simulink model "AVR_library"  (R2019b)
settings: Solver=VariableStepAuto  StartTime=0.0  StopTime=10.0  RelTol=1e-3
undefined symbols (not defined in the file or in its folder): dyn, gcbh, j, sps_rtmsupport, Tb1, Tc1
libraries: simulink x5, spsST2AModel x4, modelLibrary x3
settings Model: Creator=gdudgeon  LastModifiedBy=gdudgeon
settings SFSimCC: CustomCodeUndefinedFunction=UseInterfaceOnly

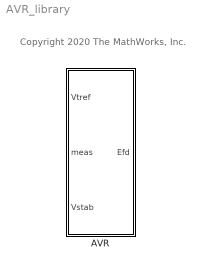
== system AVR_library ==
  note: Copyright 2020 The MathWorks, Inc.
  AVR : Subsystem  VariantControlMode=Label  Variant=on  LabelModeActiveChoice=Variant1
      settings: AttributesFormatString=%<BlockChoice>

== system AVR_library/AVR ==
  Vtref : Inport
  meas : Inport  Port=2
  Vstab : Inport  Port=3
  REXS : Subsystem  VariantControl=Variant1  mask{p=dyn.rexs_102_GAS}
      mask prompts: p "Parameters"
      mask DialogControl DescGroupVar Prompt: REXS
  ST1A : Subsystem  VariantControl=Variant2  mask{p=dyn.esst1a_102_HYDRO}
      mask prompts: p "Parameters"
      mask DialogControl DescGroupVar Prompt: ST1A
  ST4B : Subsystem  VariantControl=Variant3  mask{p=dyn.esst4b_102_STEAM}
      mask prompts: p "Parameters"
      mask DialogControl DescGroupVar Prompt: ST4B
  Efd : Outport  VectorParamsAs1DForOutWhenUnconnected=off

== system AVR_library/AVR/REXS ==
  Vtref : Inport
  meas : Inport  Port=2
  Vstab : Inport  Port=3
  Bus Selector1 : BusSelector  OutputSignals="dq0 components.Stator voltage  vd (pu),dq0 components.Stator voltage  vq (pu),dq0 components.Stator current  id (pu),dq0 components.Stator current  iq (pu),dq0 components.Field current  ifd (pu)"
  Euclidian Norm3 : Subsystem
  Euclidian Norm4 : Subsystem
  "Rotating Excitation System (Continuous) " : Subsystem  mask(PSS1A - Single Input Power System Stabilizer){Tr=p.tr, Kvp=p.kvp, Kvi=p.kvi, Vimax=p.vimax, Ta=p.ta, Tb=[p.tb1 p.tb2], Tc=[p.tc1 p.tc2], Vrrange=[p.vrmin p.vrmax], Kf=p.kf, Tf=p.tf, Tfll=[p.tf1 p.tf2], Fbf=p.fbf, Kip=p.kip, Kii=p.kii, Tp=p.tp, Kh=p.kh, Ke=p.ke, Te=p.te, Vfrange=[p.vfmin p.vfmax], Kc=p.kc, Kd=p.kd, E=[p.e1 p.e2], Se=[p.se1 p.se2], Xc=p.xc, Vcmax=p.vcmax, Kefd=p.kefd}
      mask prompts: Tr "Tr, Voltage Transducer Time Constant [s]"; Kvp "Kvp, Proportional Gain"; Kvi "Kvi, Integral Gain"; Vimax "Vimax, Input Limit [pu]"; Ta "Ta, Time Constant [s]"; Tb "Tb, Lag Time Constants [s]"; Tc "Tc, Lead Time Constants [s]"; Vrrange "[Vrmin Vrmax], Output Range [pu]"; Kf "Kf, Rate Gain"; Tf "Tf, Rate Time Constant [s]"; Tfll "[Tf1 Tf2], Lead/lag Contants [s]"; Fbf "Fbf, Feedback Signal Fl"; Kip "Kip, Regulator Proportional Gain"; Kii "Kii, Regulator Inegral Gain"; Tp "Tp, Bridge Time Constant [s]"; Kh "Kh, Voltage Controller Gain"; Ke "Ke, Exciter Proportional Constant"; Te "Te, Exciter Time Constant [s]"; Vfrange "[Vfmin Vfmax], Field Current Bounds [pu]"; Kc "Kc, Rectifier Regulation Factor [pu]"; Kd "Kd, Exciter Regulation Factor [pu]"; E "[E1 E2], Field Voltage Value Saturation"; Se "[Se1 Se2], Saturation Factor"; Xc "Xc,  Compounding Reactance [pu]"; Vcmax "Vcmax, Maximum Compounding Voltage [pu]"; Kefd "Kefd, Field Voltage Feedback"
      mask init:
      | % Extract Parameters
      | Tb1 = Tb(1);        Tb2 = Tb(2);
      | Tc1 = Tc(1);        Tc2 = Tc(2);
      | Tf1 = Tfll(1);      Tf2 = Tfll(2);
      | Vrmin = Vrrange(1); Vrmax = Vrrange(2);
      | Vfmin = Vfrange(1); Vfmax = Vfrange(2);
      mask DialogControl Container9 Prompt: Voltage Regulator
      mask DialogControl Container11 Prompt: Feedback Dynamics
      mask DialogControl Container25 Prompt: Field Current Regulator
      mask DialogControl Container29 Prompt: Rotating Exciter
      mask Display:
      | port_label('input',1,'Vref');
      | port_label('input',2,'Vt');
      | port_label('input',3,'It');
      | port_label('input',4,'Ifd');
      | port_label('input',5,'Vstab');
      | port_label('output',1,'Efd');
      | 
      | color('blue');disp('AVR/Exciter')
  Efd : Outport  VectorParamsAs1DForOutWhenUnconnected=off
  wires:
  meas/1 -> Bus Selector1/1
  "Rotating Excitation System (Continuous) "/1(Efd) -> Efd/1
  Bus Selector1/5 -> "Rotating Excitation System (Continuous) "/4(Ifd)  "<Field current  ifd (pu)>"
  Euclidian Norm3/1(y) -> "Rotating Excitation System (Continuous) "/2(Vt)  "Vt"
  Bus Selector1/2 -> Euclidian Norm3/2(u2)  "<Stator voltage  vq (pu)>"
  Bus Selector1/4 -> Euclidian Norm4/2(u2)  "<Stator current  iq (pu)>"
  Euclidian Norm4/1(y) -> "Rotating Excitation System (Continuous) "/3(It)  "It"
  Bus Selector1/3 -> Euclidian Norm4/1(u1)  "<Stator current  id (pu)>"
  Vtref/1 -> "Rotating Excitation System (Continuous) "/1(Vref)
  Bus Selector1/1 -> Euclidian Norm3/1(u1)  "<Stator voltage  vd (pu)>"
  Vstab/1 -> "Rotating Excitation System (Continuous) "/5(Vstab)

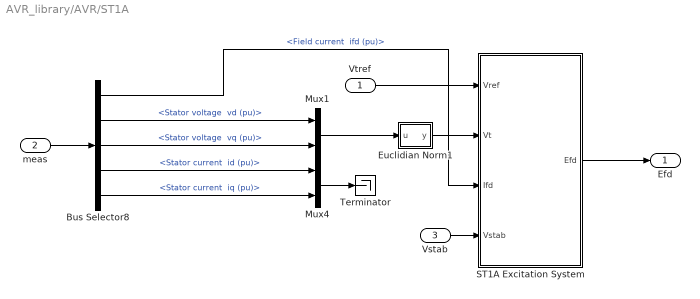
== system AVR_library/AVR/ST1A ==
  Vtref : Inport
  meas : Inport  Port=2
  Vstab : Inport  Port=3
  Bus Selector8 : BusSelector  OutputSignals="dq0 components.Field current  ifd (pu),dq0 components.Stator voltage  vd (pu),dq0 components.Stator voltage  vq (pu),dq0 components.Stator current  id (pu),dq0 components.Stator current  iq (pu)"
  Euclidian Norm1 : Subsystem
  Mux1 : Mux  Inputs=2
  Mux4 : Mux  Inputs=2
  ST1A Excitation System : Subsystem  DialogController=POWERSYS.PowerSysDialog  LoadFcn=sps_rtmsupport('LoadFcn', gcbh);  StartFcn=sps_rtmsupport('StartFcn', gcbh);  StopFcn=sps_rtmsupport('StopFcn', gcbh);  mask(ST1A Excitation System){Tr=20e-3, KaTa=[p.ka p.ta], VIminmax=[p.vimin p.vimax], VAminmax=[p.vamin p.vamax], VRminmax=[p.vrmin p.vrmax], KfTf=[p.kf p.tf], TbTc=[p.tb p.tc p.tb1 p.tc1], KLR=p.klr, ILR=p.ilr, Kc=p.kc, v0=[1 1], TsBlock=0}
      mask prompts: Tr "Low-pass filter time constant Tr(s):"; KaTa "Voltage regulator gain and time constant [Ka Ta(s)]:"; VIminmax "Voltage regulator input limits [VImin(pu) VImax(pu)]:"; VAminmax "Voltage regulator internal limits [VAmin(pu) VAmax(pu)]:"; VRminmax "Voltage regulator output limits [VRmin(pu) VRmax(pu)]:"; KfTf "Damping filter gain and time constant [Kf Tf(s)]:"; TbTc "Transient gain reduction lead and lag time constants [Tb(s) Tc(s) Tb1(s) Tc1(s)]:"; KLR "Exciter output current limiter gain KLR(pu):"; ILR "Exciter output current limit reference ILR(pu):"; Kc "Rectifier loading factor Kc(pu):"; v0 "Initial values of terminal voltage and field voltage [Vt0(pu) Efd0(pu)]:"; TsBlock "Sample time:"
      mask help: Implements a synchronous machine voltage regulator and exciter based on the IEEE type ST1A excitation system model. The output is the field voltage to apply to the Vf input of a Synchronous Machine block. Inputs and output are in p.u.
      mask init:
      | Ka = KaTa(1);
      | Ta = KaTa(2);
      | 
      | Kf = KfTf(1);
      | Tf = KfTf(2);
      | 
      | Tb = TbTc(1);
      | Tc = TbTc(2);
      settings: CopyFcn=sps_rtmsupport('CopyFcn', gcbh);  DeleteFcn=sps_rtmsupport('DeleteFcn', gcbh);  UndoDeleteFcn=sps_rtmsupport('UndoDeleteFcn', gcbh);  ModelCloseFcn=sps_rtmsupport('ModelCloseFcn', gcbh);  PreSaveFcn=sps_rtmsupport('PreSaveFcn', gcbh);  PostSaveFcn=sps_rtmsupport('PostSaveFcn', gcbh);  NameChangeFcn=sps_rtmsupport('NameChangeFcn', gcbh);  PreCopyFcn=sps_rtmsupport('PreCopyFcn', gcbh);  OpenFcn=sps_rtmsupport('OpenFcn', gcbh, []);  CloseFcn=sps_rtmsupport('CloseFcn', gcbh);  PreDeleteFcn=sps_rtmsupport('PreDeleteFcn', gcbh);
      mask Help: helpview(psbhelp);
      mask DialogControl ParameterTabVar0 Prompt: Controllers
      mask DialogControl ParameterTabVar01 Prompt: Exciter and Rectifier
      mask DialogControl ParameterTabVar012 Prompt: Initial Values
      mask Display: color('blue');disp('ST1A')
  Terminator : Terminator
  Efd : Outport  VectorParamsAs1DForOutWhenUnconnected=off
  wires:
  Mux4/1 -> Terminator/1
  ST1A Excitation System/1(Efd) -> Efd/1
  Vstab/1 -> ST1A Excitation System/4(Vstab)
  Bus Selector8/1 -> ST1A Excitation System/3(Ifd)  "<Field current  ifd (pu)>"
  Vtref/1 -> ST1A Excitation System/1(Vref)
  Bus Selector8/5 -> Mux4/2  "<Stator current  iq (pu)>"
  Bus Selector8/4 -> Mux4/1  "<Stator current  id (pu)>"
  meas/1 -> Bus Selector8/1
  Euclidian Norm1/1(y) -> ST1A Excitation System/2(Vt)
  Bus Selector8/2 -> Mux1/1  "<Stator voltage  vd (pu)>"
  Bus Selector8/3 -> Mux1/2  "<Stator voltage  vq (pu)>"
  Mux1/1 -> Euclidian Norm1/1(u)

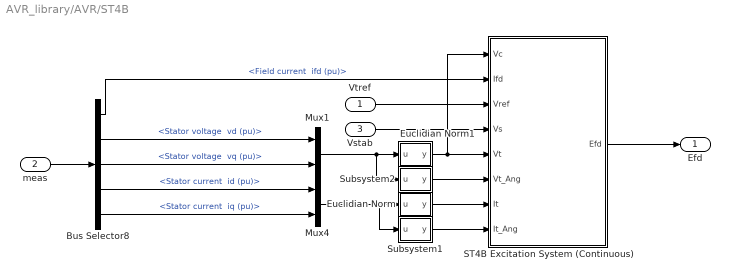
== system AVR_library/AVR/ST4B ==
  Vtref : Inport
  meas : Inport  Port=2
  Vstab : Inport  Port=3
  Bus Selector8 : BusSelector  OutputSignals="dq0 components.Field current  ifd (pu),dq0 components.Stator voltage  vd (pu),dq0 components.Stator voltage  vq (pu),dq0 components.Stator current  id (pu),dq0 components.Stator current  iq (pu)"
  Euclidian Norm : Subsystem
  Euclidian Norm1 : Subsystem
  Mux1 : Mux  Inputs=2
  Mux4 : Mux  Inputs=2
  ST4B Excitation System (Continuous) : Subsystem  mask(ST4B Excitation System){Tr=p.tr, Kpr=p.kpr, Kir=p.kir, Ta=p.ta, Vrmax=p.vrmax, Vrmin=p.vrmin, Kpm=p.kpm, Kim=p.kim, Kg=p.kg, Vmmin=p.vmmin, Vmmax=p.vmmax, Vgmax=p.vgmax, Kp=p.kp, Ki=p.ki, Angp=p.angp, Kc=p.kc, Xl=p.xl, Vbmax=p.vbmax}
      mask prompts: Tr "Voltage Transducer Time (Tr)"; Kpr "AVR Proportional Gain (Kpr)"; Kir "AVR Integral Gain (Kir)"; Ta "AVR Time Constant (Ta) [sec]"; Vrmax "Maximum AVR Output (Vrmax)"; Vrmin "Minimum AVR Output (Vrmin)"; Kpm "Inner Loop Regulator P Gain (Kpm)"; Kim "Inner Loop Regulator I gain (Kim)"; Kg "Inner Loop Feedback Gain (Kg)"; Vmmin "Inner Loop Regulator Min Output (Vmmin)"; Vmmax "Inner Loop Regulator Max Output (Vmmax)"; Vgmax "Maximum inner loop feedback gain [Vgmax(pu)]"; Kp "Potential circuit gain coefficient (Kp)"; Ki "Current circuit gain coefficient (Ki)"; Angp "Potential Source Phase Angle [Angp (rad)]"; Kc "Rectifier loading factor (Kc)"; Xl "Leakage Reactance (XL)"; Vbmax "Maximum Excitation Voltage (Vbmax)"
      mask help:
      | Implements ST4B excitation system.
      |
      | Units of parameters are in PU unless otherwise noted.
      |
      | The ST4B Excitation System block currently only has a Continuous implementation and thus cannot have a specified sample time.
      mask DialogControl Container7 Prompt: Controllers
      mask DialogControl Container5 Prompt: Exciter and Rectifier
      mask Display: color('blue');disp('ST4B')
  Subsystem1 : Subsystem
  Subsystem2 : Subsystem
  Efd : Outport  VectorParamsAs1DForOutWhenUnconnected=off
  wires:
  Mux1/1 -> Euclidian Norm1/1(u), Subsystem2/1(u)
  Bus Selector8/3 -> Mux1/2  "<Stator voltage  vq (pu)>"
  Bus Selector8/2 -> Mux1/1  "<Stator voltage  vd (pu)>"
  Vtref/1 -> ST4B Excitation System (Continuous)/3(Vref)
  Euclidian Norm/1(y) -> ST4B Excitation System (Continuous)/7(It)
  Mux4/1 -> Subsystem1/1(u), Euclidian Norm/1(u)
  Subsystem1/1(y) -> ST4B Excitation System (Continuous)/8(It_Ang)
  Euclidian Norm1/1(y) -> ST4B Excitation System (Continuous)/5(Vt), ST4B Excitation System (Continuous)/1(Vc)
  Subsystem2/1(y) -> ST4B Excitation System (Continuous)/6(Vt_Ang)
  Vstab/1 -> ST4B Excitation System (Continuous)/4(Vs)
  meas/1 -> Bus Selector8/1
  Bus Selector8/1 -> ST4B Excitation System (Continuous)/2(Ifd)  "<Field current  ifd (pu)>"
  Bus Selector8/4 -> Mux4/1  "<Stator current  id (pu)>"
  Bus Selector8/5 -> Mux4/2  "<Stator current  iq (pu)>"
  ST4B Excitation System (Continuous)/1(Efd) -> Efd/1

== system AVR_library/AVR/REXS/Euclidian Norm3 ==
  u1 : Inport
  u2 : Inport  Port=2
  Math Function : Math  Operator=square  SaturateOnIntegerOverflow=on
  Mux : Mux  Inputs=2
  Sqrt : Sqrt  SaturateOnIntegerOverflow=on
  Sum of Elements : Sum  Inputs=+
  y : Outport  VectorParamsAs1DForOutWhenUnconnected=off
  wires:
  Sum of Elements/1 -> Sqrt/1
  Math Function/1 -> Sum of Elements/1
  u1/1 -> Mux/1
  u2/1 -> Mux/2
  Mux/1 -> Math Function/1
  Sqrt/1 -> y/1

== system AVR_library/AVR/REXS/Euclidian Norm4 ==
  u1 : Inport
  u2 : Inport  Port=2
  Math Function : Math  Operator=square  SaturateOnIntegerOverflow=on
  Mux : Mux  Inputs=2
  Sqrt : Sqrt  SaturateOnIntegerOverflow=on
  Sum of Elements : Sum  Inputs=+
  y : Outport  VectorParamsAs1DForOutWhenUnconnected=off
  wires:
  Sqrt/1 -> y/1
  Mux/1 -> Math Function/1
  u2/1 -> Mux/2
  u1/1 -> Mux/1
  Math Function/1 -> Sum of Elements/1
  Sum of Elements/1 -> Sqrt/1

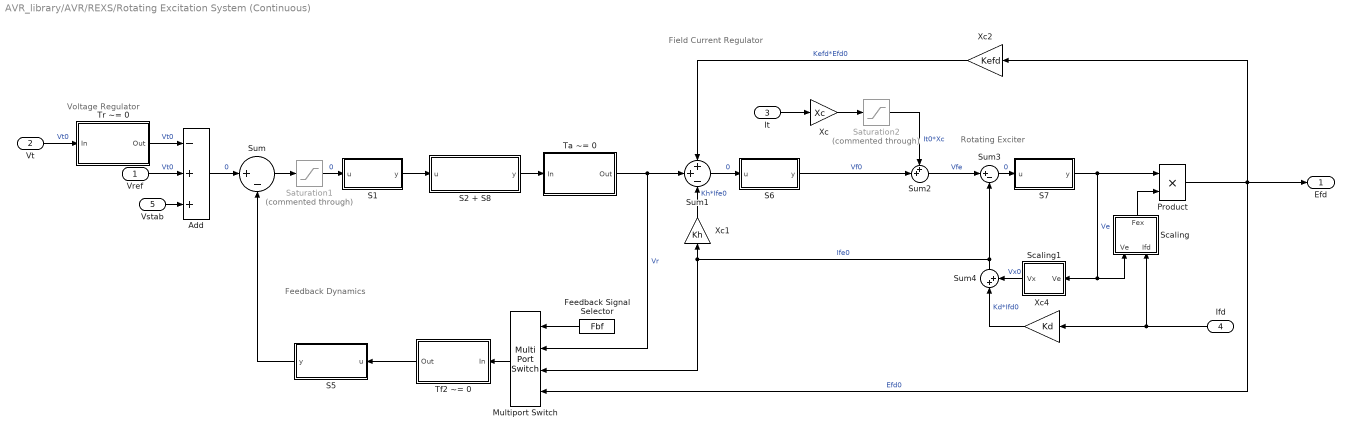
== system AVR_library/AVR/REXS/Rotating Excitation System (Continuous)  ==
  note: Field Current Regulator
  note: Feedback Dynamics
  note: Rotating Exciter
  note: Voltage Regulator
  Vref : Inport
  Vt : Inport  Port=2
  It : Inport  Port=3
  Ifd : Inport  Port=4
  Vstab : Inport  Port=5
  Add : Sum  Inputs=-++
  Feedback Signal Selector : Constant  Value=Fbf
  Multiport Switch : MultiPortSwitch  DataPortOrder=Zero-based contiguous  zeroidx=on
  Product : Product
  S1 : Subsystem
      mask Display: disp('K_{vp} + K_{vi}/s','texmode','on');
  S2 + S8 : Subsystem
      mask Display: disp('(1 + s T_{c1})(1 + s T_{c2})/(1 + s T_{b1})(1 + s T_{b2})','texmode','on');
  S5 : Subsystem
      mask Display: disp('s K_f / (1 + s T_f)','texmode','on');
  S6 : Subsystem
      mask Display: disp('K_{ip} + K_{ii}/s','texmode','on');
  S7 : Subsystem
      mask Display: disp('1/(s T_e)','texmode','on');
  Saturation1 : Saturate  Commented=through  UpperLimit=Vimax  LowerLimit=-Vimax
      settings: AttributesFormatString=|
      | %<UpperLimit>
      | %<LowerLimit>
  Saturation2 : Saturate  Commented=through  UpperLimit=Vcmax  LowerLimit=-Inf
      settings: AttributesFormatString=|
      | %<UpperLimit>
      | %<LowerLimit>
  Scaling : Subsystem
      mask Display: disp('F(I_{fd},V_e)','texmode','on');
  Scaling1 : Subsystem
      mask Display: disp('K_e + S_e','texmode','on');
  Sum : Sum  Inputs=|+-
  Sum1 : Sum  Inputs=++-
  Sum2 : Sum  Inputs=++|
  Sum3 : Sum  Inputs=|+-
  Sum4 : Sum  Inputs=|++
  Ta ~= 0 : Subsystem  VariantControl=TaNotZero
  Tf2 ~= 0 : Subsystem  VariantControl=Tf2NotZero
  Tr ~= 0 : Subsystem  VariantControl=TrNotZero
  Xc : Gain  Gain=Xc
  Xc1 : Gain  Gain=Kh
  Xc2 : Gain  Gain=Kefd
  Xc4 : Gain  Gain=Kd
  Efd : Outport  VectorParamsAs1DForOutWhenUnconnected=off
  wires:
  Vt/1 -> Tr ~= 0/1(In)  "Vt0"
  Tr ~= 0/1(Out) -> Add/1  "Vt0"
  Vref/1 -> Add/2  "Vt0"
  Vstab/1 -> Add/3
  Add/1 -> Sum/1  "0"
  Sum/1 -> Saturation1/1
  Saturation1/1 -> S1/1(u)  "0"
  S1/1(y) -> S2 + S8/1(u)
  S2 + S8/1(y) -> Ta ~= 0/1(In)
  Ta ~= 0/1(Out) -> Multiport Switch/2, Sum1/2  "Vr"
  Sum1/1 -> S6/1(u)  "0"
  S6/1(y) -> Sum2/2  "Vf0"
  Xc/1 -> Saturation2/1
  Saturation2/1 -> Sum2/1  "It0*Xc"
  Sum2/1 -> Sum3/1  "Vfe"
  Sum3/1 -> S7/1(u)  "0"
  Sum4/1 -> Xc1/1, Multiport Switch/3, Sum3/2  "Ife0"
  Xc1/1 -> Sum1/3  "Kh*Ife0"
  Xc2/1 -> Sum1/1  "Kefd*Efd0"
  Product/1 -> Xc2/1, Efd/1, Multiport Switch/4  "Efd0"
  Scaling1/1(Vx) -> Sum4/2  "Vx0"
  S7/1(y) -> Product/1, Scaling1/1(Ve), Scaling/1(Ve)  "Ve"
  Xc4/1 -> Sum4/1  "Kd*Ifd0"
  Scaling/1(Fex) -> Product/2
  Feedback Signal Selector/1 -> Multiport Switch/1
  Multiport Switch/1 -> Tf2 ~= 0/1(In)
  Tf2 ~= 0/1(Out) -> S5/1(u)
  S5/1(y) -> Sum/2
  Ifd/1 -> Xc4/1, Scaling/2(Ifd)
  It/1 -> Xc/1

== system AVR_library/AVR/ST1A/Euclidian Norm1 ==
  u : Inport
  Math Function : Math  Operator=square  SaturateOnIntegerOverflow=on
  Sqrt : Sqrt  SaturateOnIntegerOverflow=on
  Sum of Elements : Sum  Inputs=+
  y : Outport  VectorParamsAs1DForOutWhenUnconnected=off
  wires:
  u/1 -> Math Function/1
  Sqrt/1 -> y/1  "t"
  Math Function/1 -> Sum of Elements/1
  Sum of Elements/1 -> Sqrt/1

== system AVR_library/AVR/ST1A/ST1A Excitation System ==
  Vref : Inport
  Vt : Inport  Port=2
  Ifd : Inport  Port=3
  Vstab : Inport  Port=4
  Model : Subsystem  mask(Excitation System){}
  Efd : Outport  VectorParamsAs1DForOutWhenUnconnected=off
  wires:
  Model/1(Efd) -> Efd/1
  Vt/1 -> Model/2(Vt)
  Vref/1 -> Model/1(Vref)
  Ifd/1 -> Model/3(Ifd)
  Vstab/1 -> Model/4(Vstab)

== system AVR_library/AVR/ST4B/Euclidian Norm ==
  u : Inport
  Math Function : Math  Operator=square  SaturateOnIntegerOverflow=on
  Sqrt : Sqrt  SaturateOnIntegerOverflow=on
  Sum of Elements : Sum  Inputs=+
  y : Outport  VectorParamsAs1DForOutWhenUnconnected=off
  wires:
  Sum of Elements/1 -> Sqrt/1
  Math Function/1 -> Sum of Elements/1
  Sqrt/1 -> y/1  "t"
  u/1 -> Math Function/1

== system AVR_library/AVR/ST4B/Euclidian Norm1 ==
  u : Inport
  Math Function : Math  Operator=square  SaturateOnIntegerOverflow=on
  Sqrt : Sqrt  SaturateOnIntegerOverflow=on
  Sum of Elements : Sum  Inputs=+
  y : Outport  VectorParamsAs1DForOutWhenUnconnected=off
  wires:
  Sum of Elements/1 -> Sqrt/1
  Math Function/1 -> Sum of Elements/1
  Sqrt/1 -> y/1  "t"
  u/1 -> Math Function/1

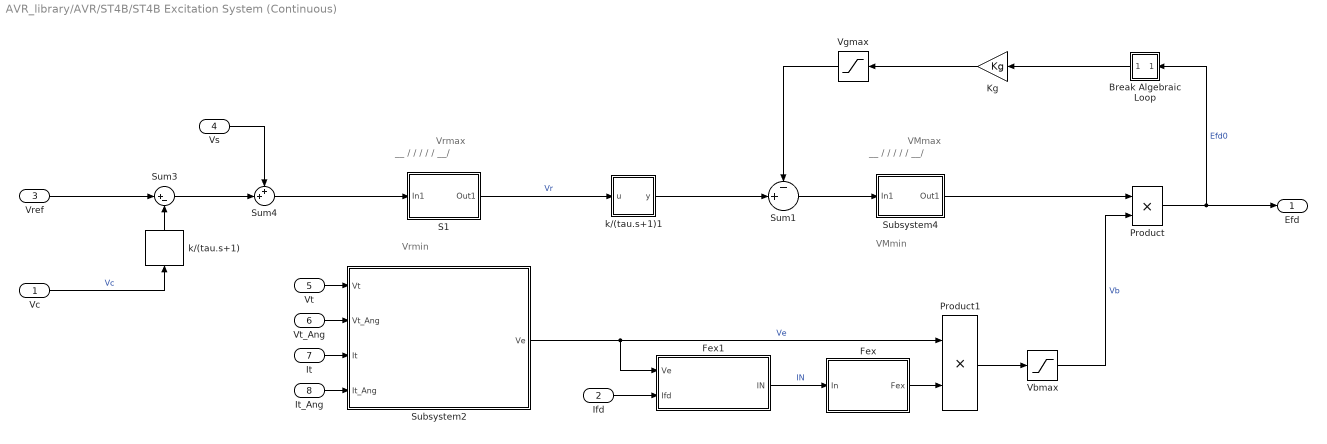
== system AVR_library/AVR/ST4B/ST4B Excitation System (Continuous) ==
  note: VMmin
  note: VMmax
  note: __
      |               /
      |             /
      |           /
      |         /
      |       /
      | __/
  note: Vrmin
  note: Vrmax
  note: __
      |               /
      |             /
      |           /
      |         /
      |       /
      | __/
  Vc : Inport
  Ifd : Inport  Port=2
  Vref : Inport  Port=3
  Vs : Inport  Port=4
  Vt : Inport  Port=5
  Vt_Ang : Inport  Port=6
  It : Inport  Port=7
  It_Ang : Inport  Port=8
  "Break Algebraic Loop " : Subsystem
      mask Display: disp('1 / (1 + s T_{pelec})','texmode','on');
  Fex : Subsystem
      mask Display: disp('Fex = f(IN)');
  Fex1 : Subsystem  mask{Kc=Kc}
      mask prompts: Kc "Exciter regulation factor, Kc(pu):"
      mask Display: disp('In = Kc*Ifd/Ve')
  Kg : Gain  Gain=Kg
  Product : Product  SaturateOnIntegerOverflow=on  RndMeth=Zero  InputSameDT=on  OutDataTypeStr=Inherit: Same as first input
  Product1 : Product  SaturateOnIntegerOverflow=on  RndMeth=Zero  InputSameDT=on  OutDataTypeStr=Inherit: Same as first input
  S1 : Subsystem
      mask Display: disp('K_{pr} + K_{ir}/s','texmode','on');
  Subsystem2 : Subsystem
      mask Display: disp('Ve = |Kp*Vt+j(Ki+Kp*XL)*It|')
  Subsystem4 : Subsystem
      mask Display: disp('K_{pm} + K_{im}/s','texmode','on');
  Sum1 : Sum  Inputs=-+|
  Sum3 : Sum  Inputs=|+-
  Sum4 : Sum  Inputs=++|
  Vbmax : Saturate  UpperLimit=Vbmax  LowerLimit=-inf
  Vgmax : Saturate  UpperLimit=Vgmax  LowerLimit=-inf
  k/(tau.s+1) : modelLibrary/k//(tau.s+1)  k=1  tau=Tr  vmax=Inf  vmin=-Inf
  k/(tau.s+1)1 : Subsystem  mask{k=1, tau=Ta, vmax=Inf, vmin=-Inf}
  Efd : Outport  VectorParamsAs1DForOutWhenUnconnected=off
  wires:
  Subsystem4/1(Out1) -> Product/1
  S1/1(Out1) -> k/(tau.s+1)1/1(u)  "Vr"
  k/(tau.s+1)1/1(y) -> Sum1/2
  "Break Algebraic Loop "/1(Out) -> Kg/1
  Vgmax/1 -> Sum1/1
  Ifd/1 -> Fex1/2(Ifd)
  It_Ang/1 -> Subsystem2/4(It_Ang)
  Fex/1(Fex) -> Product1/2
  Fex1/1(IN) -> Fex/1(In)  "IN"
  Vt_Ang/1 -> Subsystem2/2(Vt_Ang)
  Vt/1 -> Subsystem2/1(Vt)
  Product1/1 -> Vbmax/1
  Kg/1 -> Vgmax/1
  Sum1/1 -> Subsystem4/1(In1)
  Sum4/1 -> S1/1(In1)
  Subsystem2/1(Ve) -> Fex1/1(Ve), Product1/1  "Ve"
  Vbmax/1 -> Product/2  "Vb"
  It/1 -> Subsystem2/3(It)
  Product/1 -> "Break Algebraic Loop "/1(In), Efd/1  "Efd0"
  Vc/1 -> k/(tau.s+1)/1  "Vc"
  Sum3/1 -> Sum4/2
  Vs/1 -> Sum4/1
  k/(tau.s+1)/1 -> Sum3/2
  Vref/1 -> Sum3/1

== system AVR_library/AVR/ST4B/Subsystem1 ==
  u : Inport
  Demux : Demux  Outputs=2
  Divide : Product  Inputs=*/
  Trigonometric Function : Trigonometry  Operator=atan
  y : Outport  VectorParamsAs1DForOutWhenUnconnected=off
  wires:
  Divide/1 -> Trigonometric Function/1
  Trigonometric Function/1 -> y/1
  Demux/2 -> Divide/2
  u/1 -> Demux/1
  Demux/1 -> Divide/1

== system AVR_library/AVR/ST4B/Subsystem2 ==
  u : Inport
  Demux : Demux  Outputs=2
  Divide : Product  Inputs=*/
  Trigonometric Function : Trigonometry  Operator=atan
  y : Outport  VectorParamsAs1DForOutWhenUnconnected=off
  wires:
  Divide/1 -> Trigonometric Function/1
  Trigonometric Function/1 -> y/1
  Demux/2 -> Divide/2
  u/1 -> Demux/1
  Demux/1 -> Divide/1

== system AVR_library/AVR/REXS/Rotating Excitation System (Continuous) /S1 ==
  u : Inport
  Gain1 : Gain  Gain=Kvi
  Gain7 : Gain  Gain=Kvp
  Integrator : Integrator
  Sum : Sum  Inputs=|++
  y : Outport  InitialOutput=0  VectorParamsAs1DForOutWhenUnconnected=off
  wires:
  u/1 -> Gain1/1, Gain7/1
  Gain1/1 -> Integrator/1
  Gain7/1 -> Sum/1
  Integrator/1 -> Sum/2
  Sum/1 -> y/1

== system AVR_library/AVR/REXS/Rotating Excitation System (Continuous) /S2 + S8 ==
  u : Inport
  S2 : Subsystem  VariantControlMode=Label  Variant=on  LabelModeActiveChoice=Tb1NotZero
      mask Display: disp('(1 + s T_{c1}) / (1 + s T_{b1})','texmode','on');
  S8 : Subsystem  VariantControlMode=Label  Variant=on  LabelModeActiveChoice=Tb2NotZero
      mask Display: disp('(1 + s T_{c2}) / (1 + s T_{b2})','texmode','on');
  y : Outport  InitialOutput=0  VectorParamsAs1DForOutWhenUnconnected=off
  wires:
  S8/1(Out) -> y/1
  S2/1(Out) -> S8/1(In)
  u/1 -> S2/1(In)

== system AVR_library/AVR/REXS/Rotating Excitation System (Continuous) /S5 ==
  u : Inport
  Gain : Gain  Gain=1/Tf
  Gain1 : Gain  Gain=Kf
  Integrator : Integrator
  Sum : Sum  Inputs=|+-
  y : Outport  InitialOutput=0  VectorParamsAs1DForOutWhenUnconnected=off
  wires:
  Gain/1 -> Gain1/1, Integrator/1
  Integrator/1 -> Sum/2
  Sum/1 -> Gain/1
  u/1 -> Sum/1
  Gain1/1 -> y/1

== system AVR_library/AVR/REXS/Rotating Excitation System (Continuous) /S6 ==
  u : Inport
  Gain1 : Gain  Gain=Kii
  Gain7 : Gain  Gain=Kip
  Integrator : Integrator
  Sum : Sum  Inputs=|++
  y : Outport  InitialOutput=0  VectorParamsAs1DForOutWhenUnconnected=off
  wires:
  Sum/1 -> y/1
  Integrator/1 -> Sum/2
  Gain7/1 -> Sum/1
  Gain1/1 -> Integrator/1
  u/1 -> Gain7/1, Gain1/1

== system AVR_library/AVR/REXS/Rotating Excitation System (Continuous) /S7 ==
  u : Inport
  Gain1 : Gain  Gain=1/Te
  Integrator : Integrator  InitialCondition=1  LimitOutput=on  LowerSaturationLimit=0
  y : Outport  InitialOutput=0  VectorParamsAs1DForOutWhenUnconnected=off
  wires:
  Integrator/1 -> y/1
  Gain1/1 -> Integrator/1
  u/1 -> Gain1/1

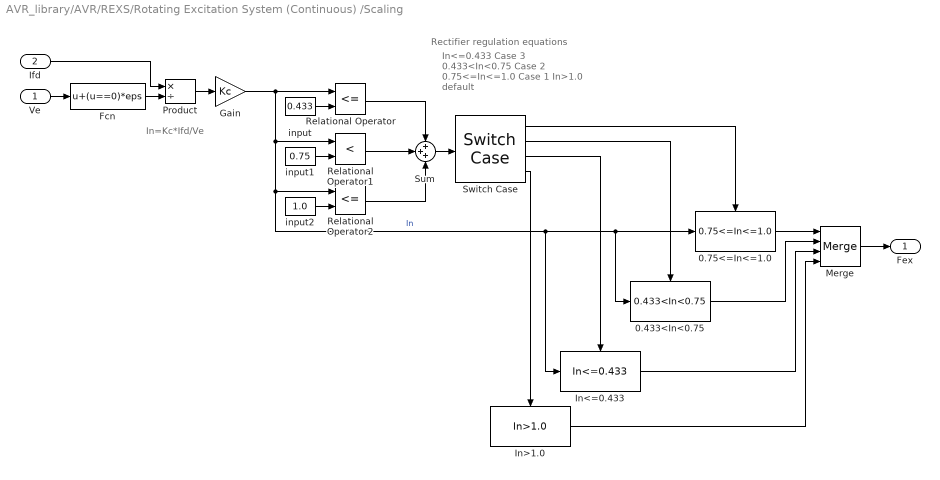
== system AVR_library/AVR/REXS/Rotating Excitation System (Continuous) /Scaling ==
  note: In=Kc*Ifd/Ve
  note: Rectifier regulation equations
  note: In<=0.433        Case 3
      | 0.433<In<0.75 Case 2
      | 0.75<=In<=1.0 Case 1
      | In>1.0               default
  Ve : Inport
  Ifd : Inport  Port=2
  0.433<In<0.75 : spsST2AModel/Continuous/Rectifier/0.433<In<0.75  SystemSampleTime=-1  Latency=0  AutoFrameSizeCalculation=off
      settings: SourceProductName=Simscape Electrical  SourceProductBaseCode=PS
  0.75<=In<=1.0 : spsST2AModel/Continuous/Rectifier/0.75<=In<=1.0  SystemSampleTime=-1  Latency=0  AutoFrameSizeCalculation=off
      settings: SourceProductName=Simscape Electrical  SourceProductBaseCode=PS
  Fcn : Fcn  Expr=u+(u==0)*eps
  Gain : Gain  Gain=Kc  SaturateOnIntegerOverflow=on  OutDataTypeStr=Inherit: Same as input  ParamDataTypeStr=Inherit: Same as input
  In<=0.433 : spsST2AModel/Continuous/Rectifier/In<=0.433  SystemSampleTime=-1  Latency=0  AutoFrameSizeCalculation=off
      settings: SourceProductName=Simscape Electrical  SourceProductBaseCode=PS
  In>1.0 : spsST2AModel/Continuous/Rectifier/In>1.0  SystemSampleTime=-1  Latency=0  AutoFrameSizeCalculation=off
      settings: SourceProductName=Simscape Electrical  SourceProductBaseCode=PS
  Merge : Merge  Inputs=4
  Product : Product  Inputs=*/  SaturateOnIntegerOverflow=on  RndMeth=Zero  InputSameDT=on  OutDataTypeStr=Inherit: Same as first input
  Relational Operator : RelationalOperator  Operator=<=  RndMeth=Nearest  InputSameDT=on
  Relational Operator1 : RelationalOperator  Operator=<  RndMeth=Nearest  InputSameDT=on
  Relational Operator2 : RelationalOperator  Operator=<=  RndMeth=Nearest  InputSameDT=on
  Sum : Sum  Inputs=+++  AccumDataTypeStr=double  OutDataTypeStr=double  SaturateOnIntegerOverflow=on  InputSameDT=on
  Switch Case : SwitchCase  CaseConditions={1 2 3}
  input : Constant  Value=0.433
  input1 : Constant  Value=0.75
  input2 : Constant  Value=1.0
  Fex : Outport  VectorParamsAs1DForOutWhenUnconnected=off
  wires:
  input/1 -> Relational Operator/2
  Switch Case/4 -> In>1.0/Action
  Switch Case/3 -> In<=0.433/Action
  Switch Case/2 -> 0.433<In<0.75/Action
  Switch Case/1 -> 0.75<=In<=1.0/Action
  Sum/1 -> Switch Case/1
  Relational Operator2/1 -> Sum/3
  Relational Operator/1 -> Sum/1
  Relational Operator1/1 -> Sum/2
  input2/1 -> Relational Operator2/2
  input1/1 -> Relational Operator1/2
  In<=0.433/1 -> Merge/3
  In>1.0/1 -> Merge/4
  0.433<In<0.75/1 -> Merge/2
  0.75<=In<=1.0/1 -> Merge/1
  Merge/1 -> Fex/1
  Gain/1 -> Relational Operator/1, Relational Operator1/1, In<=0.433/1, 0.75<=In<=1.0/1, 0.433<In<0.75/1, Relational Operator2/1  "In"
  Product/1 -> Gain/1
  Ifd/1 -> Product/1
  Fcn/1 -> Product/2
  Ve/1 -> Fcn/1

== system AVR_library/AVR/REXS/Rotating Excitation System (Continuous) /Scaling1 ==
  Ve : Inport
  1-D Lookup Table : Lookup_n-D  NumberOfTableDimensions=1  BreakpointsForDimension1=[0 E(1) E(2)]  Table=[0 Se(1) Se(2)]  InternalRulePriority=Speed  RndMeth=Simplest  InputSameDT=on
  Product1 : Product  RndMeth=Zero
  Sum : Sum  Inputs=++|
  Xc4 : Gain  Gain=Ke
  Vx : Outport  VectorParamsAs1DForOutWhenUnconnected=off
  wires:
  Sum/1 -> Vx/1
  Ve/1 -> Xc4/1, 1-D Lookup Table/1, Product1/1
  1-D Lookup Table/1 -> Product1/2  "Se[Ve]"
  Product1/1 -> Sum/2
  Xc4/1 -> Sum/1

== system AVR_library/AVR/REXS/Rotating Excitation System (Continuous) /Ta ~= 0 ==
  In : Inport
  1/Ta : Gain  Gain=1/Ta
  Integrator : Integrator  InitialCondition=0.5  LimitOutput=on  UpperSaturationLimit=Vrmax  LowerSaturationLimit=Vrmin
  Sum : Sum  Inputs=|+-
  Out : Outport  InitialOutput=0  VectorParamsAs1DForOutWhenUnconnected=off
  wires:
  Integrator/1 -> Out/1, Sum/2
  In/1 -> Sum/1
  1/Ta/1 -> Integrator/1
  Sum/1 -> 1/Ta/1

== system AVR_library/AVR/REXS/Rotating Excitation System (Continuous) /Tf2 ~= 0 ==
  In : Inport
  Gain : Gain  Gain=1/Tf2
  Gain1 : Gain  Gain=Tf1
  Integrator : Integrator
  Sum : Sum  Inputs=|+-
  Sum1 : Sum  Inputs=++|
  Out : Outport  InitialOutput=0  VectorParamsAs1DForOutWhenUnconnected=off
  wires:
  In/1 -> Sum/1
  Sum1/1 -> Out/1
  Gain/1 -> Gain1/1, Integrator/1
  Sum/1 -> Gain/1
  Integrator/1 -> Sum1/2, Sum/2
  Gain1/1 -> Sum1/1

== system AVR_library/AVR/REXS/Rotating Excitation System (Continuous) /Tr ~= 0 ==
  In : Inport
  1/Tr : Gain  Gain=1/Tr
  Integrator : Integrator
  Sum : Sum  Inputs=|+-
  Out : Outport  InitialOutput=0  VectorParamsAs1DForOutWhenUnconnected=off
  wires:
  Integrator/1 -> Out/1, Sum/2
  In/1 -> Sum/1
  1/Tr/1 -> Integrator/1
  Sum/1 -> 1/Tr/1

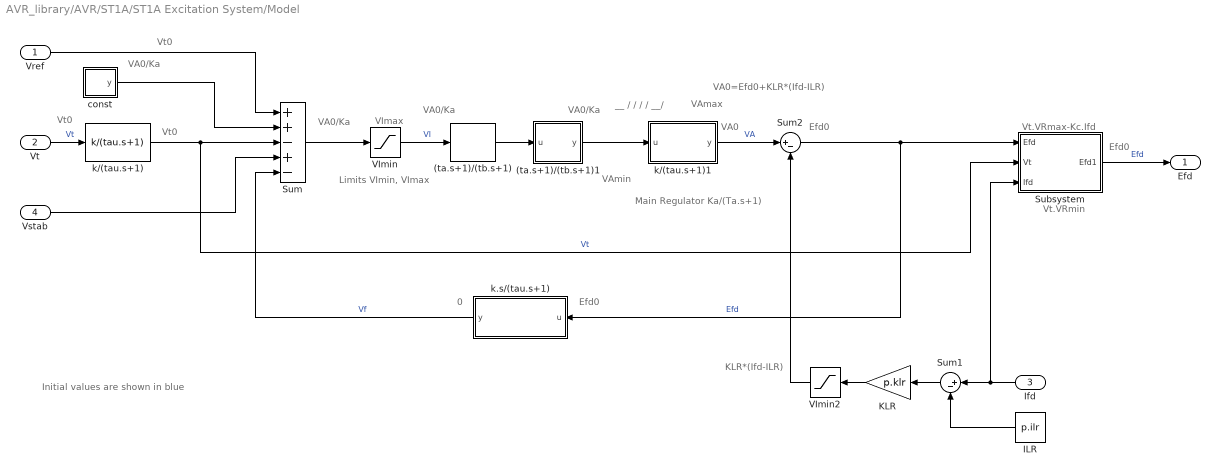
== system AVR_library/AVR/ST1A/ST1A Excitation System/Model ==
  note: Vt0
  note: VA0
  note: VA0=Efd0+KLR*(Ifd-ILR)
  note: KLR*(Ifd-ILR)
  note: VA0/Ka
  note: VAmin
  note: VAmax
  note: Limits VImin, VImax
  note: __
      |              /
      |           /
      |         /
      |       /
      | __/
  note: Vt0
  note: Initial values are shown in blue
  note: VImax
  note: Main Regulator
      | Ka/(Ta.s+1)
  note: Vt.VRmax-Kc.Ifd
  note: Vt0
  note: 0
  note: Efd0
  note: VA0/Ka
  note: Vt.VRmin
  note: VA0/Ka
  note: VA0/Ka
  note: Efd0
  note: Efd0
  Vref : Inport
  Vt : Inport  Port=2
  Ifd : Inport  Port=3
  Vstab : Inport  Port=4
  (ta.s+1)/(tb.s+1) : modelLibrary/(ta.s+1)//(tb.s+1)  ta=Tc  tb=Tb
  (ta.s+1)/(tb.s+1)1 : Subsystem  mask{ta=Tc1, tb=Tb1}
      mask prompts: ta "numerator tau (ta)"; tb "denominator tau  (tb)"
  ILR : Constant  Value=p.ilr
  KLR : Gain  Gain=p.klr  SaturateOnIntegerOverflow=on  OutDataTypeStr=Inherit: Same as input  ParamDataTypeStr=Inherit: Same as input
  Subsystem : Subsystem
      mask Display: plot([0.15 0.85],[.5 .5],[.5 .5],[0.05 0.95],0.15+0.7*[0 .25 .75 1],0.05+0.9*[.25 .25 .75 .75]);
  Sum : Sum  Inputs=++-+-  SaturateOnIntegerOverflow=on  InputSameDT=on  OutDataTypeStr=Inherit: Same as first input
  Sum1 : Sum  Inputs=|+-  SaturateOnIntegerOverflow=on  InputSameDT=on  OutDataTypeStr=Inherit: Same as first input
  Sum2 : Sum  Inputs=|+-  SaturateOnIntegerOverflow=on  InputSameDT=on  OutDataTypeStr=Inherit: Same as first input
  VImin : Saturate  UpperLimit=p.vimax  LowerLimit=p.vimin
  VImin2 : Saturate  UpperLimit=inf  LowerLimit=0
  const : Subsystem
  k.s/(tau.s+1) : Subsystem  mask{k=Kf, tau=Tf}
  k/(tau.s+1) : modelLibrary/k//(tau.s+1)  k=1  tau=p.tr  vmax=Inf  vmin=-Inf
  k/(tau.s+1)1 : Subsystem  mask{k=p.ka, tau=p.ta, vmax=p.vamax, vmin=p.vamin}
  Efd : Outport  VectorParamsAs1DForOutWhenUnconnected=off
  wires:
  (ta.s+1)/(tb.s+1)/1 -> (ta.s+1)/(tb.s+1)1/1(u)
  const/1(y) -> Sum/2
  Vstab/1 -> Sum/4
  VImin/1 -> (ta.s+1)/(tb.s+1)/1  "VI"
  k.s/(tau.s+1)/1(y) -> Sum/5  "Vf"
  VImin2/1 -> Sum2/2
  k/(tau.s+1)/1 -> Subsystem/2(Vt), Sum/3  "Vt"
  Vref/1 -> Sum/1
  KLR/1 -> VImin2/1
  (ta.s+1)/(tb.s+1)1/1(y) -> k/(tau.s+1)1/1(u)
  Sum2/1 -> Subsystem/1(Efd), k.s/(tau.s+1)/1(u)  "Efd"
  ILR/1 -> Sum1/2
  Sum1/1 -> KLR/1
  Sum/1 -> VImin/1
  k/(tau.s+1)1/1(y) -> Sum2/1  "VA"
  Vt/1 -> k/(tau.s+1)/1  "Vt"
  Subsystem/1(Efd1) -> Efd/1  "Efd"
  Ifd/1 -> Subsystem/3(Ifd), Sum1/1

== system AVR_library/AVR/ST4B/ST4B Excitation System (Continuous)/Break Algebraic Loop  ==
  In : Inport
  1/Tau : Gain  Gain=1/1e-3
  Integrator : Integrator  InitialCondition=1
  Sum : Sum  Inputs=|+-
  Out : Outport  InitialOutput=0  VectorParamsAs1DForOutWhenUnconnected=off
  wires:
  Sum/1 -> 1/Tau/1
  1/Tau/1 -> Integrator/1
  In/1 -> Sum/1
  Integrator/1 -> Sum/2, Out/1

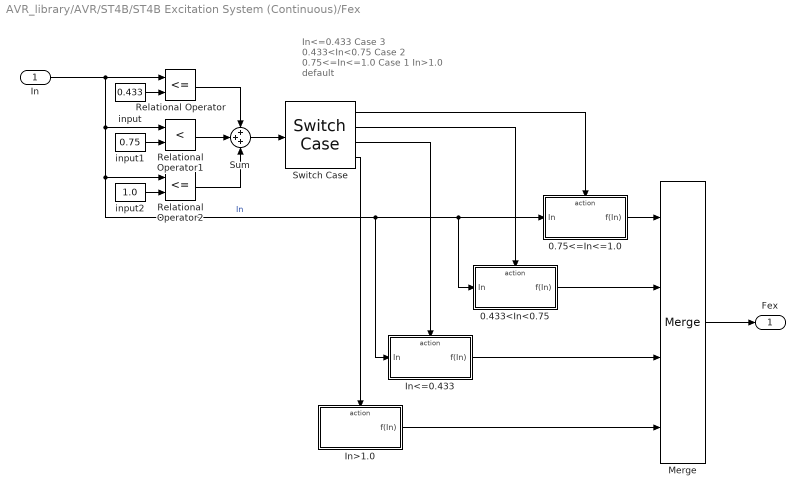
== system AVR_library/AVR/ST4B/ST4B Excitation System (Continuous)/Fex ==
  note: In<=0.433        Case 3
      | 0.433<In<0.75 Case 2
      | 0.75<=In<=1.0 Case 1
      | In>1.0               default
  In : Inport
  0.433<In<0.75 : Subsystem  TreatAsAtomicUnit=on
  0.75<=In<=1.0 : Subsystem  TreatAsAtomicUnit=on
  In<=0.433 : Subsystem  TreatAsAtomicUnit=on
  In>1.0 : Subsystem  TreatAsAtomicUnit=on
  Merge : Merge  Inputs=4
  Relational Operator : RelationalOperator  Operator=<=  RndMeth=Nearest  InputSameDT=on
  Relational Operator1 : RelationalOperator  Operator=<  RndMeth=Nearest  InputSameDT=on
  Relational Operator2 : RelationalOperator  Operator=<=  RndMeth=Nearest  InputSameDT=on
  Sum : Sum  Inputs=+++  AccumDataTypeStr=double  OutDataTypeStr=double  SaturateOnIntegerOverflow=on  InputSameDT=on
  Switch Case : SwitchCase  CaseConditions={1 2 3}
  input : Constant  Value=0.433
  input1 : Constant  Value=0.75
  input2 : Constant  Value=1.0
  Fex : Outport  VectorParamsAs1DForOutWhenUnconnected=off
  wires:
  input/1 -> Relational Operator/2
  Switch Case/4 -> In>1.0/Action
  Switch Case/3 -> In<=0.433/Action
  Switch Case/2 -> 0.433<In<0.75/Action
  Switch Case/1 -> 0.75<=In<=1.0/Action
  Sum/1 -> Switch Case/1
  Relational Operator2/1 -> Sum/3
  Relational Operator/1 -> Sum/1
  Relational Operator1/1 -> Sum/2
  input2/1 -> Relational Operator2/2
  input1/1 -> Relational Operator1/2
  In<=0.433/1(f(In)) -> Merge/3
  In>1.0/1(f(In)) -> Merge/4
  0.433<In<0.75/1(f(In)) -> Merge/2
  0.75<=In<=1.0/1(f(In)) -> Merge/1
  In/1 -> Relational Operator/1, Relational Operator1/1, In<=0.433/1(In), 0.433<In<0.75/1(In), 0.75<=In<=1.0/1(In), Relational Operator2/1  "In"
  Merge/1 -> Fex/1

== system AVR_library/AVR/ST4B/ST4B Excitation System (Continuous)/Fex1 ==
  Ve : Inport
  Ifd : Inport  Port=2
  Fcn : Fcn  Expr=u+(u==0)*eps
  Gain : Gain  Gain=Kc  SaturateOnIntegerOverflow=on  OutDataTypeStr=Inherit: Same as input  ParamDataTypeStr=Inherit: Same as input
  Product : Product  Inputs=*/  SaturateOnIntegerOverflow=on  RndMeth=Zero  InputSameDT=on  OutDataTypeStr=Inherit: Same as first input
  IN : Outport  VectorParamsAs1DForOutWhenUnconnected=off
  wires:
  Gain/1 -> IN/1  "In"
  Ve/1 -> Fcn/1
  Fcn/1 -> Product/2
  Ifd/1 -> Product/1
  Product/1 -> Gain/1

== system AVR_library/AVR/ST4B/ST4B Excitation System (Continuous)/S1 ==
  In1 : Inport
  Gain2 : Gain  Gain=Kpr
  Gain3 : Gain  Gain=Kir
  Integrator (Anti-windup) : Subsystem
      mask Display: dpoly([1],[1 0],'s')
  Saturation1 : Saturate  UpperLimit=Vrmax  LowerLimit=Vrmin
  Sum2 : Sum  Inputs=|++
  Out1 : Outport  VectorParamsAs1DForOutWhenUnconnected=off
  wires:
  Saturation1/1 -> Out1/1
  Sum2/1 -> Saturation1/1, Integrator (Anti-windup)/2(ctrlOutput1)
  Gain2/1 -> Sum2/1
  Integrator (Anti-windup)/1(Out2) -> Sum2/2
  In1/1 -> Gain2/1, Gain3/1
  Gain3/1 -> Integrator (Anti-windup)/1(u)

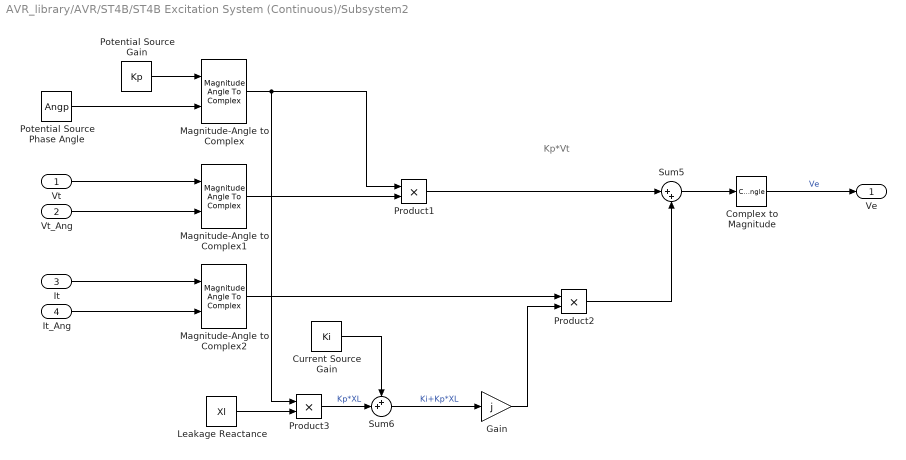
== system AVR_library/AVR/ST4B/ST4B Excitation System (Continuous)/Subsystem2 ==
  note: Kp*Vt
  Vt : Inport
  Vt_Ang : Inport  Port=2
  It : Inport  Port=3
  It_Ang : Inport  Port=4
  Complex to Magnitude : ComplexToMagnitudeAngle  Output=Magnitude
  Current Source Gain : Constant  Value=Ki
  Gain : Gain  Gain=j
  Leakage Reactance : Constant  Value=Xl
  Magnitude-Angle to Complex : MagnitudeAngleToComplex
  Magnitude-Angle to Complex1 : MagnitudeAngleToComplex
  Magnitude-Angle to Complex2 : MagnitudeAngleToComplex
  Potential Source Gain : Constant  Value=Kp
  Potential Source Phase Angle : Constant  Value=Angp
  Product1 : Product  SaturateOnIntegerOverflow=on  RndMeth=Zero  InputSameDT=on  OutDataTypeStr=Inherit: Same as first input
  Product2 : Product  SaturateOnIntegerOverflow=on  RndMeth=Zero  InputSameDT=on  OutDataTypeStr=Inherit: Same as first input
  Product3 : Product  SaturateOnIntegerOverflow=on  RndMeth=Zero  InputSameDT=on  OutDataTypeStr=Inherit: Same as first input
  Sum5 : Sum  Inputs=|++
  Sum6 : Sum  Inputs=++|
  Ve : Outport  VectorParamsAs1DForOutWhenUnconnected=off
  wires:
  It_Ang/1 -> Magnitude-Angle to Complex2/2
  Vt_Ang/1 -> Magnitude-Angle to Complex1/2
  It/1 -> Magnitude-Angle to Complex2/1
  Gain/1 -> Product2/2
  Sum6/1 -> Gain/1  "Ki+Kp*XL"
  Current Source Gain/1 -> Sum6/1
  Product3/1 -> Sum6/2  "Kp*XL"
  Leakage Reactance/1 -> Product3/2
  Magnitude-Angle to Complex/1 -> Product1/1, Product3/1
  Complex to Magnitude/1 -> Ve/1  "Ve"
  Vt/1 -> Magnitude-Angle to Complex1/1
  Sum5/1 -> Complex to Magnitude/1
  Product2/1 -> Sum5/2
  Product1/1 -> Sum5/1
  Potential Source Gain/1 -> Magnitude-Angle to Complex/1
  Magnitude-Angle to Complex1/1 -> Product1/2
  Potential Source Phase Angle/1 -> Magnitude-Angle to Complex/2
  Magnitude-Angle to Complex2/1 -> Product2/1

== system AVR_library/AVR/ST4B/ST4B Excitation System (Continuous)/Subsystem4 ==
  In1 : Inport
  Gain2 : Gain  Gain=Kpm
  Gain3 : Gain  Gain=Kim
  Integrator (Anti-windup) : Subsystem
      mask Display: dpoly([1],[1 0],'s')
  Saturation1 : Saturate  UpperLimit=Vmmax  LowerLimit=Vmmin
  Sum2 : Sum  Inputs=|++
  Out1 : Outport  VectorParamsAs1DForOutWhenUnconnected=off
  wires:
  Sum2/1 -> Saturation1/1, Integrator (Anti-windup)/2(ctrlOutput1)
  In1/1 -> Gain3/1, Gain2/1
  Integrator (Anti-windup)/1(Out2) -> Sum2/2
  Gain2/1 -> Sum2/1
  Saturation1/1 -> Out1/1
  Gain3/1 -> Integrator (Anti-windup)/1(u)

== system AVR_library/AVR/ST4B/ST4B Excitation System (Continuous)/k//(tau.s+1)1 ==
  u : Inport
  1/(taus+1) : Subsystem  mask{tau=tau, vmax=vmax, vmin=vmin}
      mask prompts: tau "Time Constant"
      mask init:
      | h = gcbh;
      | 
      | qq = get(h,'MaskValues');
      | 
      | if eval(qq{1}) == 0
      |     
      |     set(h,'Commented','through');
      |     
      | else
      |     
      |     set(h,'Commented','off');
      |     
      | end
  k : Gain  Gain=k
  y : Outport  VectorParamsAs1DForOutWhenUnconnected=off
  wires:
  k/1 -> 1/(taus+1)/1(u)
  u/1 -> k/1
  1/(taus+1)/1(y) -> y/1

== system AVR_library/AVR/REXS/Rotating Excitation System (Continuous) /S2 + S8/S2 ==
  In : Inport
  Tb1 = 0 : Subsystem  VariantControl=Tb1Zero
  Tb1 ~= 0 : Subsystem  VariantControl=Tb1NotZero
  Out : Outport  VectorParamsAs1DForOutWhenUnconnected=off

== system AVR_library/AVR/REXS/Rotating Excitation System (Continuous) /S2 + S8/S8 ==
  In : Inport
  Tb2 = 0 : Subsystem  VariantControl=Tb2Zero
  Tb2 ~= 0 : Subsystem  VariantControl=Tb2NotZero
  Out : Outport  VectorParamsAs1DForOutWhenUnconnected=off

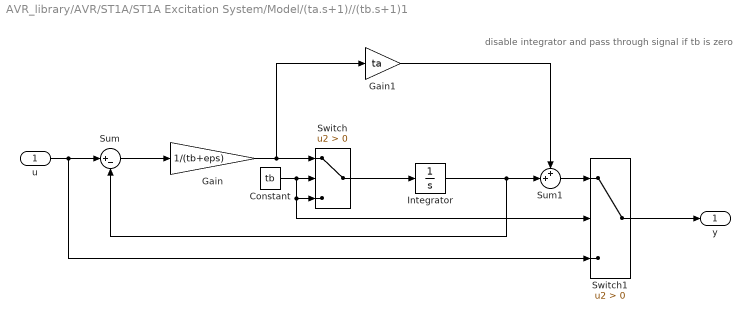
== system AVR_library/AVR/ST1A/ST1A Excitation System/Model/(ta.s+1)//(tb.s+1)1 ==
  note: disable integrator and pass through signal if tb is zero
  u : Inport
  Constant : Constant  Value=tb
  Gain : Gain  Gain=1/(tb+eps)
  Gain1 : Gain  Gain=ta
  Integrator : Integrator
  Sum : Sum  Inputs=|+-
  Sum1 : Sum  Inputs=++|
  Switch : Switch  Criteria=u2 > Threshold
  Switch1 : Switch  Criteria=u2 > Threshold
  y : Outport  VectorParamsAs1DForOutWhenUnconnected=off
  wires:
  Sum/1 -> Gain/1
  Gain/1 -> Switch/1, Gain1/1
  Gain1/1 -> Sum1/1
  Integrator/1 -> Sum1/2, Sum/2
  u/1 -> Switch1/3, Sum/1
  Constant/1 -> Switch1/2, Switch/3, Switch/2
  Switch/1 -> Integrator/1
  Sum1/1 -> Switch1/1
  Switch1/1 -> y/1

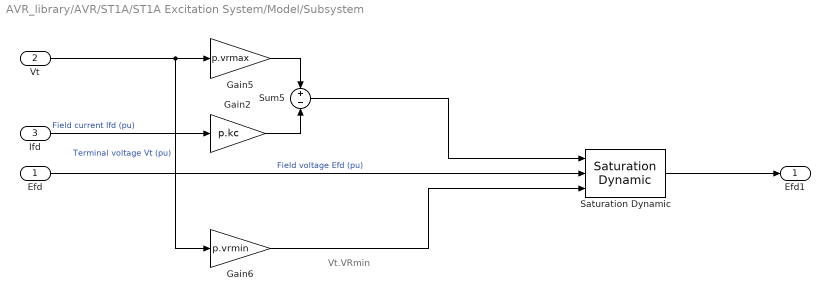
== system AVR_library/AVR/ST1A/ST1A Excitation System/Model/Subsystem ==
  note: Vt.VRmin
  Efd : Inport
  Vt : Inport  Port=2
  Ifd : Inport  Port=3
  Gain2 : Gain  Gain=p.kc  SaturateOnIntegerOverflow=on  OutDataTypeStr=Inherit: Same as input  ParamDataTypeStr=Inherit: Same as input
  Gain5 : Gain  Gain=p.vrmax  SaturateOnIntegerOverflow=on  OutDataTypeStr=Inherit: Same as input  ParamDataTypeStr=Inherit: Same as input
  Gain6 : Gain  Gain=p.vrmin  SaturateOnIntegerOverflow=on  OutDataTypeStr=Inherit: Same as input  ParamDataTypeStr=Inherit: Same as input
  Saturation Dynamic : simulink/Discontinuities/Saturation Dynamic  OutMin=[]  OutMax=[]  OutDataTypeStr=Inherit: Same as second input  OutDataType=fixdt(1, 16)  OutScaling=2^-10  DoSatur=off
  Sum5 : Sum  Inputs=+-  SaturateOnIntegerOverflow=on  InputSameDT=on  OutDataTypeStr=Inherit: Same as first input
  Efd1 : Outport  VectorParamsAs1DForOutWhenUnconnected=off
  wires:
  Gain6/1 -> Saturation Dynamic/3
  Sum5/1 -> Saturation Dynamic/1
  Saturation Dynamic/1 -> Efd1/1
  Vt/1 -> Gain5/1, Gain6/1  "Terminal voltage Vt (pu)"
  Gain5/1 -> Sum5/1
  Efd/1 -> Saturation Dynamic/2  "Field voltage Efd (pu)"
  Ifd/1 -> Gain2/1  "Field current Ifd (pu)"
  Gain2/1 -> Sum5/2

== system AVR_library/AVR/ST1A/ST1A Excitation System/Model/const ==
  Constant : Constant  Value=0
  Integrator : Integrator
  y : Outport  VectorParamsAs1DForOutWhenUnconnected=off
  wires:
  Integrator/1 -> y/1
  Constant/1 -> Integrator/1

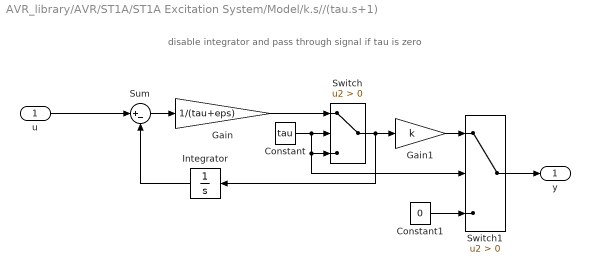
== system AVR_library/AVR/ST1A/ST1A Excitation System/Model/k.s//(tau.s+1) ==
  note: disable integrator and pass through signal if tau is zero
  u : Inport
  Constant : Constant  Value=tau
  Constant1 : Constant  Value=0
  Gain : Gain  Gain=1/(tau+eps)
  Gain1 : Gain  Gain=k
  Integrator : Integrator
  Sum : Sum  Inputs=|+-
  Switch : Switch  Criteria=u2 > Threshold
  Switch1 : Switch  Criteria=u2 > Threshold
  y : Outport  VectorParamsAs1DForOutWhenUnconnected=off
  wires:
  Constant1/1 -> Switch1/3
  Integrator/1 -> Sum/2
  u/1 -> Sum/1
  Sum/1 -> Gain/1
  Constant/1 -> Switch1/2, Switch/3, Switch/2
  Gain/1 -> Switch/1
  Switch/1 -> Integrator/1, Gain1/1
  Switch1/1 -> y/1
  Gain1/1 -> Switch1/1

== system AVR_library/AVR/ST1A/ST1A Excitation System/Model/k//(tau.s+1)1 ==
  u : Inport
  1/(taus+1) : Subsystem  mask{tau=tau, vmax=vmax, vmin=vmin}
      mask prompts: tau "Time Constant"
  k : Gain  Gain=k
  y : Outport  VectorParamsAs1DForOutWhenUnconnected=off
  wires:
  1/(taus+1)/1(y) -> y/1
  u/1 -> k/1
  k/1 -> 1/(taus+1)/1(u)

== system AVR_library/AVR/ST4B/ST4B Excitation System (Continuous)/Fex/0.433<In<0.75 ==
  In : Inport
  Action Port : ActionPort  InitializeStates=reset
  Math Function : Math  Operator=square  SaturateOnIntegerOverflow=on
  Math Function1 : Math  Operator=sqrt  SaturateOnIntegerOverflow=on
  Sum : Sum  Inputs=+-|  SaturateOnIntegerOverflow=on  InputSameDT=on  OutDataTypeStr=Inherit: Same as first input
  input2 : Constant  Value=0.75
  f(In) : Outport  VectorParamsAs1DForOutWhenUnconnected=off
  wires:
  Sum/1 -> Math Function1/1
  input2/1 -> Sum/1
  Math Function/1 -> Sum/2
  In/1 -> Math Function/1
  Math Function1/1 -> f(In)/1

== system AVR_library/AVR/ST4B/ST4B Excitation System (Continuous)/Fex/0.75<=In<=1.0 ==
  In : Inport
  Action Port : ActionPort  InitializeStates=reset
  Gain : Gain  Gain=1.732  SaturateOnIntegerOverflow=on  OutDataTypeStr=Inherit: Same as input  ParamDataTypeStr=Inherit: Same as input
  Sum : Sum  Inputs=+-|  SaturateOnIntegerOverflow=on  InputSameDT=on  OutDataTypeStr=Inherit: Same as first input
  input2 : Constant  Value=1.0
  f(In) : Outport  VectorParamsAs1DForOutWhenUnconnected=off
  wires:
  In/1 -> Sum/2
  input2/1 -> Sum/1
  Sum/1 -> Gain/1
  Gain/1 -> f(In)/1

== system AVR_library/AVR/ST4B/ST4B Excitation System (Continuous)/Fex/In<=0.433 ==
  In : Inport
  Action Port : ActionPort  InitializeStates=reset
  Gain : Gain  Gain=0.577  SaturateOnIntegerOverflow=on  OutDataTypeStr=Inherit: Same as input  ParamDataTypeStr=Inherit: Same as input
  Sum : Sum  Inputs=+-|  SaturateOnIntegerOverflow=on  InputSameDT=on  OutDataTypeStr=Inherit: Same as first input
  input2 : Constant  Value=1.0
  f(In) : Outport  VectorParamsAs1DForOutWhenUnconnected=off
  wires:
  In/1 -> Gain/1
  Gain/1 -> Sum/2
  input2/1 -> Sum/1
  Sum/1 -> f(In)/1

== system AVR_library/AVR/ST4B/ST4B Excitation System (Continuous)/Fex/In>1.0 ==
  Action Port : ActionPort  InitializeStates=reset
  input2 : Constant  Value=0
  f(In) : Outport  InitialOutput=0  VectorParamsAs1DForOutWhenUnconnected=off
  wires:
  input2/1 -> f(In)/1

== system AVR_library/AVR/ST4B/ST4B Excitation System (Continuous)/S1/Integrator (Anti-windup) ==
  u : Inport
  ctrlOutput1 : Inport  Port=2
  Compare To Constant : simulink/Logic and Bit Operations/Compare To Constant  relop=>=  const=Vrmax  OutDataTypeStr=boolean
  Compare To Constant1 : simulink/Logic and Bit Operations/Compare To Constant  relop=<=  const=Vrmin  OutDataTypeStr=boolean
  Constant : Constant  Value=0
  Integrator : Integrator
  Logical Operator : Logic  Operator=OR  AllPortsSameDT=off  OutDataTypeStr=boolean
  Switch : Switch  Criteria=u2 > Threshold
  Out2 : Outport  VectorParamsAs1DForOutWhenUnconnected=off
  wires:
  Compare To Constant1/1 -> Logical Operator/2
  Compare To Constant/1 -> Logical Operator/1
  ctrlOutput1/1 -> Compare To Constant/1, Compare To Constant1/1
  Logical Operator/1 -> Switch/2
  Integrator/1 -> Out2/1
  Switch/1 -> Integrator/1
  u/1 -> Switch/3
  Constant/1 -> Switch/1

== system AVR_library/AVR/ST4B/ST4B Excitation System (Continuous)/Subsystem4/Integrator (Anti-windup) ==
  u : Inport
  ctrlOutput1 : Inport  Port=2
  Compare To Constant : simulink/Logic and Bit Operations/Compare To Constant  relop=>=  const=Vmmax  OutDataTypeStr=boolean
  Compare To Constant1 : simulink/Logic and Bit Operations/Compare To Constant  relop=<=  const=Vmmin  OutDataTypeStr=boolean
  Constant : Constant  Value=0
  Integrator : Integrator  InitialCondition=1
  Logical Operator : Logic  Operator=OR  AllPortsSameDT=off  OutDataTypeStr=boolean
  Switch : Switch  Criteria=u2 > Threshold
  Out2 : Outport  VectorParamsAs1DForOutWhenUnconnected=off
  wires:
  Compare To Constant1/1 -> Logical Operator/2
  Compare To Constant/1 -> Logical Operator/1
  ctrlOutput1/1 -> Compare To Constant/1, Compare To Constant1/1
  Logical Operator/1 -> Switch/2
  Constant/1 -> Switch/1
  u/1 -> Switch/3
  Switch/1 -> Integrator/1
  Integrator/1 -> Out2/1

== system AVR_library/AVR/ST4B/ST4B Excitation System (Continuous)/k//(tau.s+1)1/1//(taus+1) ==
  note: disable integrator and pass through signal if tau is zero
  u : Inport
  Constant : Constant  Value=tau
  Gain1 : Gain  Gain=1/(tau+eps)  SaturateOnIntegerOverflow=on  OutDataTypeStr=Inherit: Same as input  ParamDataTypeStr=Inherit: Same as input
  Integrator : Integrator  LimitOutput=on  UpperSaturationLimit=vmax  LowerSaturationLimit=vmin
  Sum : Sum  Inputs=|+-  SaturateOnIntegerOverflow=on  InputSameDT=on  OutDataTypeStr=Inherit: Same as first input
  Switch : Switch  Criteria=u2 > Threshold
  Switch1 : Switch  Criteria=u2 > Threshold
  y : Outport  VectorParamsAs1DForOutWhenUnconnected=off
  wires:
  u/1 -> Switch1/3, Sum/1
  Sum/1 -> Gain1/1
  Integrator/1 -> Sum/2, Switch1/1
  Constant/1 -> Switch/3, Switch1/2, Switch/2
  Gain1/1 -> Switch/1
  Switch/1 -> Integrator/1
  Switch1/1 -> y/1

== system AVR_library/AVR/REXS/Rotating Excitation System (Continuous) /S2 + S8/S2/Tb1 = 0 ==
  In : Inport
  Out : Outport  VectorParamsAs1DForOutWhenUnconnected=off
  wires:
  In/1 -> Out/1

== system AVR_library/AVR/REXS/Rotating Excitation System (Continuous) /S2 + S8/S2/Tb1 ~= 0 ==
  In : Inport
  Gain : Gain  Gain=1/Tb1
  Gain1 : Gain  Gain=Tc1
  Integrator : Integrator
  Sum : Sum  Inputs=|+-
  Sum1 : Sum  Inputs=++|
  Out : Outport  InitialOutput=0  VectorParamsAs1DForOutWhenUnconnected=off
  wires:
  In/1 -> Sum/1
  Sum1/1 -> Out/1
  Gain/1 -> Gain1/1, Integrator/1
  Sum/1 -> Gain/1
  Integrator/1 -> Sum1/2, Sum/2
  Gain1/1 -> Sum1/1

== system AVR_library/AVR/REXS/Rotating Excitation System (Continuous) /S2 + S8/S8/Tb2 = 0 ==
  In : Inport
  Out : Outport  VectorParamsAs1DForOutWhenUnconnected=off
  wires:
  In/1 -> Out/1

== system AVR_library/AVR/REXS/Rotating Excitation System (Continuous) /S2 + S8/S8/Tb2 ~= 0 ==
  In : Inport
  Gain : Gain  Gain=1/Tb2
  Gain1 : Gain  Gain=Tc2
  Integrator : Integrator
  Sum : Sum  Inputs=|+-
  Sum1 : Sum  Inputs=++|
  Out : Outport  InitialOutput=0  VectorParamsAs1DForOutWhenUnconnected=off
  wires:
  In/1 -> Sum/1
  Sum1/1 -> Out/1
  Gain/1 -> Gain1/1, Integrator/1
  Sum/1 -> Gain/1
  Integrator/1 -> Sum1/2, Sum/2
  Gain1/1 -> Sum1/1

== system AVR_library/AVR/ST1A/ST1A Excitation System/Model/k//(tau.s+1)1/1//(taus+1) ==
  note: disable integrator and pass through signal if tau is zero
  u : Inport
  Constant : Constant  Value=tau
  Gain1 : Gain  Gain=1/(tau+eps)  SaturateOnIntegerOverflow=on  OutDataTypeStr=Inherit: Same as input  ParamDataTypeStr=Inherit: Same as input
  Integrator : Integrator  LimitOutput=on  UpperSaturationLimit=vmax  LowerSaturationLimit=vmin
  Sum : Sum  Inputs=|+-  SaturateOnIntegerOverflow=on  InputSameDT=on  OutDataTypeStr=Inherit: Same as first input
  Switch : Switch  Criteria=u2 > Threshold
  Switch1 : Switch  Criteria=u2 > Threshold
  y : Outport  VectorParamsAs1DForOutWhenUnconnected=off
  wires:
  Switch1/1 -> y/1
  Switch/1 -> Integrator/1
  Gain1/1 -> Switch/1
  Constant/1 -> Switch/2, Switch1/2, Switch/3
  Integrator/1 -> Switch1/1, Sum/2
  Sum/1 -> Gain1/1
  u/1 -> Sum/1, Switch1/3
